simulink model "sim_4_newnew"  (R2015b)
settings: Solver=ode45  StartTime=0  StopTime=700  FixedStep=1e-3  RelTol=1e-4
undefined symbols (not defined in the file or in its folder): A, alpha_nc, alpha_nw, B, currentCoeffMatrix, D, E, f, H, h, K2, K3, K4, Kd_surge, Kd_sway, Kd_yaw, Ki_surge, Ki_sway, Ki_yaw, Kp_surge, Kp_sway, Kp_yaw, M_inverse, mu, N_freq, P0, Par, phi, Q, R, S, Sim, T, T_pinv, TA_sampling_time, thrusterPositionX, thrusterPositionY, thrusters, thrustersInitialAlpha, U_mean_c, U_mean_w, windCoeffMatrix, x0
libraries: simulink_extras x15, simulink x10, marine_gnc x5
(part 1 of 2)
settings Model: Creator=torstebo  LastModifiedBy=ShivJeet
settings SolverCC: MaxConsecutiveMinStep=3  SolverJacobianMethodControl=FullPerturbation  ZeroCrossControl=DisableAll  ZeroCrossAlgorithm=Adaptive
settings DataIOCC: Decimation=10  InitialState=xFinal  LimitDataPoints=off  SaveFormat=StructureWithTime  SaveOutput=off  InspectSignalLogs=on  VisualizeSimOutput=off  SaveTime=off
settings OptimizationCC: AccelVerboseBuild=on
settings DebuggingCC: AlgebraicLoopMsg=error  UnderspecifiedInitializationDetection=Classic  MergeDetectMultiDrivingBlocksExec=none  SolverPrmCheckMsg=warning  StateNameClashWarn=warning
settings HardwareCC: ProdBitPerPointer=32  ProdLargestAtomicFloat=None  ProdIntDivRoundTo=Undefined  ProdEndianess=Unspecified  ProdWordSize=32  ProdHWDeviceType=32-bit Generic
settings GRTTargetCC: GeneratePreprocessorConditionals=Disable all
settings ConfigComp: CovModelRefEnable=Off  CovSFcnEnable=off

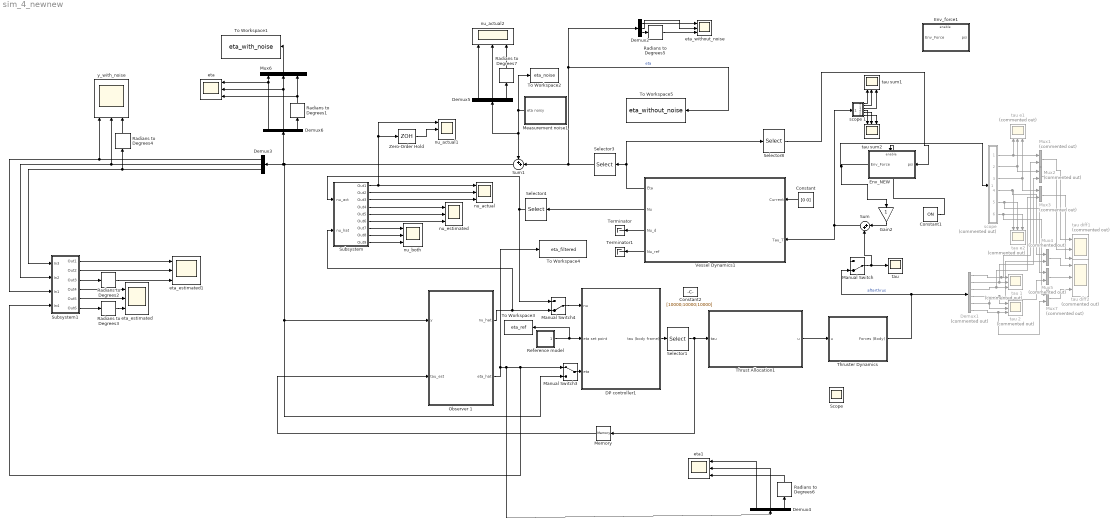
== system sim_4_newnew ==
  Constant : Constant  Value=[0 0]
  Constant1 : Constant  Value=ON
  Constant2 : Constant  Value=[10000;10000;10000]
  DP controller1 : Subsystem
  Demux1 : Demux  Commented=on  Outputs=6
  Demux{2..6} (5 alike) : Demux  Outputs=3
  Env_NEW : Subsystem
  Env_force1 : Subsystem
  Gain2 : Gain
  Manual Switch : ManualSwitch  CurrentSetting=0
  Manual Switch3 : ManualSwitch
  Manual Switch4 : ManualSwitch  CurrentSetting=0
  Measurement noise1 : Subsystem  mask{noise=on}
      mask prompts: noise "Use measurement noise"
  Memory : Memory  InheritSampleTime=on
  Mux{1..5,7} (6 alike) : Mux  Commented=on  Inputs=2
  Mux6 : Mux  Inputs=3
  Observer 1 : Subsystem
  Radians to Degrees{1..7} (7 alike) : simulink_extras/Transformations/Radians to Degrees
  Reference model : Subsystem
  Scope : Scope
  Selector1 : Selector  InputPortWidth=6  IndexOptions=Index vector (dialog)  Indices=[1 2 6]  OutputSizes=1
  Selector3 : Selector  InputPortWidth=6  IndexOptions=Index vector (dialog)  Indices=[1 2 6]  OutputSizes=1
  Selector4 : Selector  InputPortWidth=6  IndexOptions=Index vector (dialog)  Indices=[1 2 6]  OutputSizes=1
  Selector8 : Selector  InputPortWidth=6  IndexOptions=Index vector (dialog)  Indices=[6]  OutputSizes=1
  Subsystem : Subsystem
  Subsystem1 : Subsystem
  Sum : Sum  Inputs=|++
  Sum1 : Sum  Inputs=++|
  Terminator : Terminator
  Terminator1 : Terminator
  Thrust Allocation1 : Subsystem
  Thruster Dynamics : Subsystem  SystemSampleTime=TA_sampling_time  mask{wt=2, thrusterfault=off}
      mask prompts: wt "Thrusters Time constant"; thrusterfault "Thruster #3 fault?"
  To Workspace1 : ToWorkspace  VariableName=eta_with_noise  SaveFormat=Timeseries  SampleTime=-1
  To Workspace2 : ToWorkspace  VariableName=eta_noise  SaveFormat=Timeseries  SampleTime=-1
  To Workspace3 : ToWorkspace  VariableName=eta_ref  SaveFormat=Timeseries  SampleTime=-1
  To Workspace4 : ToWorkspace  VariableName=eta_filtered  SaveFormat=Timeseries  SampleTime=-1
  To Workspace5 : ToWorkspace  VariableName=eta_without_noise  SaveFormat=Timeseries  SampleTime=-1
  Vessel Dynamics1 : Subsystem
      mask Display:
      | image(imread('Files/supply.jpg'))
      | color('black'); port_label('output', 1, 'eta')
      | color('black'); port_label('output', 2, 'nu')
      | color('black'); port_label('output', 3, 'nu_d')
      | color('black'); port_label('output', 4, 'nu_ref')
      | color('black'); port_label('input', 1, 'nu_c')
      | color('black'); port_label('input', 2, 'tau')
  Zero-Order Hold : ZeroOrderHold  SampleTime=0.1
  eta : Scope  NumInputPorts=3
  eta1 : Scope  NumInputPorts=3
  eta_estimated : Scope  NumInputPorts=3
  eta_estimated1 : Scope  NumInputPorts=3
  eta_without_noise : Scope  NumInputPorts=3
  nu_actual : Scope  NumInputPorts=3
  nu_actual1 : Scope  NumInputPorts=3
  nu_actual2 : Scope  NumInputPorts=3
  "nu_both " : Scope  NumInputPorts=3
  nu_estimated : Scope  NumInputPorts=3
  "scope " : Subsystem  Commented=on
  scope 1 : Subsystem
  "tau " : Scope
  tau 1 : Scope  Commented=on  NumInputPorts=3
  tau 2 : Scope  Commented=on  NumInputPorts=3
  tau diff1 : Scope  Commented=on  NumInputPorts=3
  tau diff2 : Scope  Commented=on  NumInputPorts=3
  tau e1 : Scope  Commented=on  NumInputPorts=3
  tau e2 : Scope  Commented=on  NumInputPorts=3
  tau sum1 : Scope  NumInputPorts=3
  tau sum2 : Scope  NumInputPorts=3
  y_with_noise : Scope  NumInputPorts=3
  wires:
  Vessel Dynamics1/2(Nu) -> Selector4/1
  Constant/1 -> Vessel Dynamics1/1(Current)
  Reference model/1(Set-point) -> DP controller1/2(eta set point), To Workspace3/1
  Vessel Dynamics1/3(Nu_d) -> Terminator/1
  Thrust Allocation1/1(u) -> Thruster Dynamics/1(u)
  Vessel Dynamics1/4(Nu_ref) -> Terminator1/1
  Thruster Dynamics/1(Forces (Body)) -> Manual Switch/2, Demux1/1  "afterthrus"
  Demux6/3 -> Radians to Degrees1/1
  Radians to Degrees1/1 -> eta/3, Mux6/3
  Demux6/2 -> eta/2, Mux6/2
  Demux6/1 -> eta/1, Mux6/1
  Mux6/1 -> To Workspace1/1
  Vessel Dynamics1/1(Eta) -> Selector3/1, Selector8/1
  Selector8/1 -> Env_NEW/1(psi)
  Sum/1 -> scope 1/1(In1), Vessel Dynamics1/2(Tau_T)
  Manual Switch/1 -> "tau "/1, Sum/2
  Demux1/1 -> Mux1/2, tau 1/1
  Demux1/2 -> Mux2/2, tau 1/2
  Demux1/3 -> Mux3/2, tau 1/3
  Demux1/4 -> Mux4/2, tau 2/1
  Demux1/5 -> tau 2/2, Mux5/2
  Demux1/6 -> Mux7/2, tau 2/3
  Env_NEW/1(Env_Force) -> Gain2/1, "scope "/1(In1)
  "scope "/1(Out1) -> Mux1/1, tau e1/1
  "scope "/3(Out3) -> Mux3/1, tau e1/3
  "scope "/4(Out4) -> Mux4/1, tau e2/1
  "scope "/5(Out5) -> Mux5/1, tau e2/2
  "scope "/6(Out6) -> Mux7/1, tau e2/3
  scope 1/1(Out1) -> tau sum1/1
  scope 1/2(Out2) -> tau sum1/2
  scope 1/3(Out3) -> tau sum1/3
  scope 1/4(Out4) -> tau sum2/1
  scope 1/5(Out5) -> tau sum2/2
  scope 1/6(Out6) -> tau sum2/3
  Mux1/1 -> tau diff1/1
  "scope "/2(Out2) -> tau e1/2, Mux2/1
  Mux2/1 -> tau diff1/2
  Mux3/1 -> tau diff1/3
  Mux4/1 -> tau diff2/1
  Mux5/1 -> tau diff2/2
  Mux7/1 -> tau diff2/3
  Demux2/1 -> eta_without_noise/1
  Demux2/2 -> eta_without_noise/2
  Demux3/1 -> Subsystem1/3(In1), y_with_noise/1
  Demux3/2 -> Subsystem1/2(In2), y_with_noise/2
  Demux3/3 -> Subsystem1/1(In3), Radians to Degrees4/1
  Manual Switch4/1 -> DP controller1/1(nu)
  Observer 1/2(eta_hat) -> To Workspace4/1, Demux4/1, Subsystem1/4(In4), Manual Switch3/1
  Manual Switch3/1 -> DP controller1/3(eta)
  Selector4/1 -> Manual Switch4/1, Subsystem/1(nu_act)
  Sum1/1 -> Demux6/1, Demux3/1, Manual Switch3/2, Observer 1/1(y)
  Selector3/1 -> Demux2/1, To Workspace5/1, Sum1/2  "eta"
  Memory/1 -> Observer 1/2(tau_est)
  Subsystem/1(Out1) -> Zero-Order Hold/1, nu_actual1/1, nu_actual/1
  Subsystem/2(Out2) -> nu_actual/2
  Subsystem/3(Out3) -> nu_actual/3
  Subsystem/4(Out4) -> nu_estimated/1
  Subsystem/5(Out5) -> nu_estimated/2
  Subsystem/6(Out6) -> nu_estimated/3
  Subsystem/7(Out7) -> "nu_both "/1
  Subsystem/8(Out8) -> "nu_both "/2
  Subsystem/9(Out9) -> "nu_both "/3
  Subsystem1/1(Out1) -> eta_estimated1/1
  Subsystem1/2(Out2) -> eta_estimated1/2
  Subsystem1/3(Out3) -> Radians to Degrees2/1
  Subsystem1/4(Out4) -> eta_estimated/1
  Subsystem1/5(Out5) -> eta_estimated/2
  Subsystem1/6(Out6) -> Radians to Degrees3/1
  Radians to Degrees2/1 -> eta_estimated1/3
  Radians to Degrees3/1 -> eta_estimated/3
  Radians to Degrees4/1 -> y_with_noise/3
  Gain2/1 -> Sum/1
  Demux2/3 -> Radians to Degrees5/1
  Radians to Degrees5/1 -> eta_without_noise/3
  Demux4/3 -> Radians to Degrees6/1
  Radians to Degrees6/1 -> eta1/3
  Demux4/2 -> eta1/2
  Demux4/1 -> eta1/1
  Constant1/1 -> Env_NEW/Enable
  Observer 1/1(nu_hat) -> Subsystem/2(nu_hat), Manual Switch4/2
  Zero-Order Hold/1 -> nu_actual1/2
  Demux5/3 -> Radians to Degrees7/1
  Demux5/1 -> nu_actual2/1
  Measurement noise1/1(eta noisy) -> Demux5/1, Sum1/1, To Workspace2/1
  Demux5/2 -> nu_actual2/2
  Radians to Degrees7/1 -> nu_actual2/3
  DP controller1/1(tau (body frame)) -> Selector1/1
  Selector1/1 -> Thrust Allocation1/1(tau), Memory/1

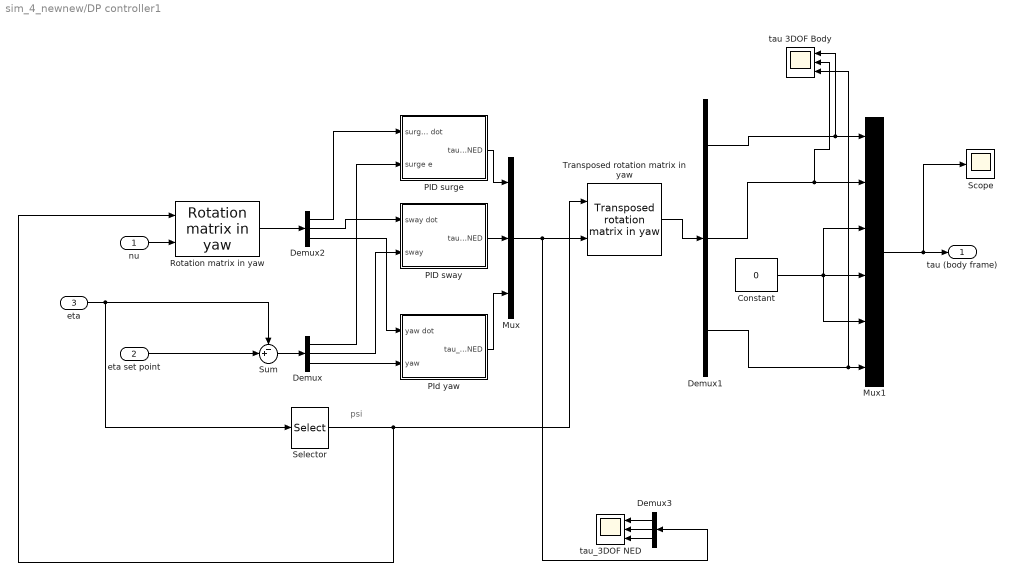
== system sim_4_newnew/DP controller1 ==
  note: psi
  nu : Inport
  eta set point : Inport  Port=2
  eta : Inport  Port=3
  Constant : Constant  Value=0
  Demux{,1..3} (4 alike) : Demux  Outputs=3
  Mux : Mux  Inputs=3
  Mux1 : Mux  Inputs=6
  PID surge : Subsystem
  PID sway : Subsystem
  "PId yaw " : Subsystem
  "Rotation matrix in yaw " : marine_gnc/Models/ Kinematics/Rotation matrix in yaw 
  Scope : Scope
  Selector : Selector  InputPortWidth=3  IndexOptions=Index vector (dialog)  Indices=3  OutputSizes=1
  Sum : Sum  Inputs=-+|
  Transposed rotation matrix in yaw : marine_gnc/Models/ Kinematics/Transposed rotation  matrix in yaw
  tau 3DOF Body : Scope  NumInputPorts=3
  tau_3DOF NED : Scope  NumInputPorts=3
  tau (body frame) : Outport
  wires:
  Sum/1 -> Demux/1
  eta/1 -> Sum/1, Selector/1
  eta set point/1 -> Sum/2
  Demux2/1 -> PID surge/1(surge dot)
  Demux/1 -> PID surge/2(surge e)
  Demux2/2 -> PID sway/1(sway dot)
  Demux2/3 -> "PId yaw "/1(yaw dot)
  Demux/2 -> PID sway/2(sway)
  Demux/3 -> "PId yaw "/2(yaw)
  "PId yaw "/1(tau_yaw_NED) -> Mux/3
  PID surge/1(tau_surge_NED) -> Mux/1
  PID sway/1(tau_sway_NED) -> Mux/2
  nu/1 -> "Rotation matrix in yaw "/2
  Selector/1 -> Transposed rotation matrix in yaw/1, "Rotation matrix in yaw "/1
  "Rotation matrix in yaw "/1 -> Demux2/1
  Constant/1 -> Mux1/3, Mux1/4, Mux1/5
  Transposed rotation matrix in yaw/1 -> Demux1/1
  Demux1/1 -> tau 3DOF Body/1, Mux1/1
  Demux1/2 -> tau 3DOF Body/2, Mux1/2
  Demux1/3 -> tau 3DOF Body/3, Mux1/6
  Mux1/1 -> Scope/1, tau (body frame)/1
  Demux3/1 -> tau_3DOF NED/1
  Demux3/2 -> tau_3DOF NED/2
  Demux3/3 -> tau_3DOF NED/3
  Mux/1 -> Transposed rotation matrix in yaw/2, Demux3/1

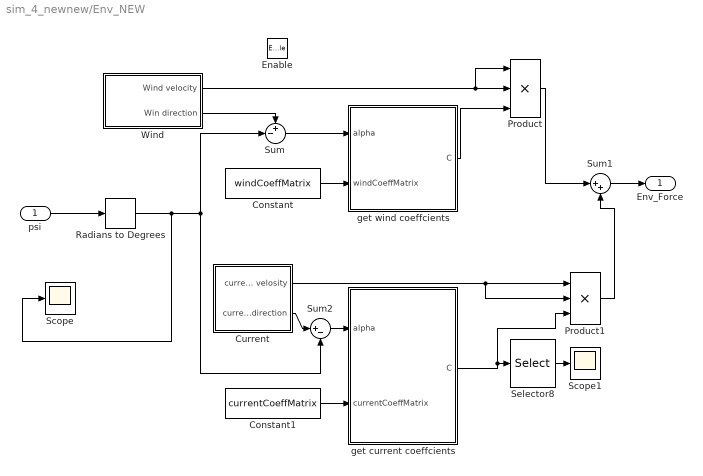
== system sim_4_newnew/Env_NEW ==
  psi : Inport
  Enable : EnablePort
  Constant : Constant  Value=windCoeffMatrix
  Constant1 : Constant  Value=currentCoeffMatrix
  Current : Subsystem
  Product : Product  Inputs=3  RndMeth=Zero
  Product1 : Product  Inputs=3  RndMeth=Zero
  Radians to Degrees : simulink_extras/Transformations/Radians to Degrees
  Scope : Scope
  Scope1 : Scope
  Selector8 : Selector  InputPortWidth=6  IndexOptions=Index vector (dialog)  Indices=[2]  OutputSizes=1
  Sum : Sum  Inputs=+-|
  Sum1 : Sum  Inputs=|++
  Sum2 : Sum  Inputs=|+-
  Wind : Subsystem
  get current coeffcients : MATLAB Function  TreatAsAtomicUnit=on
  get wind coeffcients : MATLAB Function  TreatAsAtomicUnit=on
  Env_Force : Outport
  wires:
  Wind/1(Wind velocity) -> Product/1, Product/2
  Wind/2(Win direction) -> Sum/1
  psi/1 -> Radians to Degrees/1
  Sum1/1 -> Env_Force/1
  Current/1(current velosity) -> Product1/2, Product1/1
  Radians to Degrees/1 -> Scope/1, Sum/2, Sum2/2
  Current/2(current direction) -> Sum2/1
  Sum2/1 -> get current coeffcients/1(alpha)
  get current coeffcients/1(C) -> Product1/3, Selector8/1
  Sum/1 -> get wind coeffcients/1(alpha)
  get wind coeffcients/1(C) -> Product/3
  Product1/1 -> Sum1/2
  Product/1 -> Sum1/1
  Selector8/1 -> Scope1/1
  Constant/1 -> get wind coeffcients/2(windCoeffMatrix)
  Constant1/1 -> get current coeffcients/2(currentCoeffMatrix)

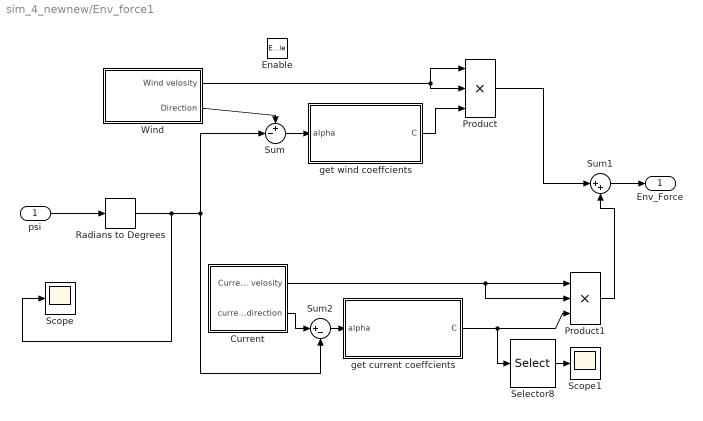
== system sim_4_newnew/Env_force1 ==
  psi : Inport
  Enable : EnablePort
  Current : Subsystem
  Product : Product  Inputs=3  RndMeth=Zero
  Product1 : Product  Inputs=3  RndMeth=Zero
  Radians to Degrees : simulink_extras/Transformations/Radians to Degrees
  Scope : Scope
  Scope1 : Scope
  Selector8 : Selector  InputPortWidth=6  IndexOptions=Index vector (dialog)  Indices=[2]  OutputSizes=1
  Sum : Sum  Inputs=+-|
  Sum1 : Sum  Inputs=|++
  Sum2 : Sum  Inputs=|+-
  Wind : Subsystem
  get current coeffcients : MATLAB Function  TreatAsAtomicUnit=on
  get wind coeffcients : MATLAB Function  TreatAsAtomicUnit=on
  Env_Force : Outport
  wires:
  Wind/1(Wind velosity) -> Product/1, Product/2
  Wind/2(Direction) -> Sum/1
  psi/1 -> Radians to Degrees/1
  Sum1/1 -> Env_Force/1
  Current/1(Current velosity) -> Product1/2, Product1/1
  Radians to Degrees/1 -> Scope/1, Sum/2, Sum2/2
  Current/2(current direction) -> Sum2/1
  Sum2/1 -> get current coeffcients/1(alpha)
  get current coeffcients/1(C) -> Selector8/1, Product1/3
  Sum/1 -> get wind coeffcients/1(alpha)
  get wind coeffcients/1(C) -> Product/3
  Product1/1 -> Sum1/2
  Product/1 -> Sum1/1
  Selector8/1 -> Scope1/1

== system sim_4_newnew/Measurement noise1 ==
  Band-Limited White Noise : simulink/Sources/Band-Limited White Noise  Cov="[0.003  0.003  0.0001]"  Ts=1/10  seed=[23341 10000 89564]
  Demux : Demux  Outputs=3
  Gain : Gain  Gain=noise
  Mux : Mux  Inputs=3
  Transfer Fcn : TransferFcn  Numerator=[10]  Denominator=[1 10]
  Transfer Fcn1 : TransferFcn  Numerator=[10]  Denominator=[1 10]
  Transfer Fcn2 : TransferFcn  Numerator=[10]  Denominator=[1 10]
  eta noisy : Outport
  wires:
  Gain/1 -> Demux/1
  Demux/3 -> Transfer Fcn2/1
  Demux/2 -> Transfer Fcn/1
  Demux/1 -> Transfer Fcn1/1
  Band-Limited White Noise/1 -> Gain/1
  Transfer Fcn2/1 -> Mux/3
  Transfer Fcn/1 -> Mux/2
  Transfer Fcn1/1 -> Mux/1
  Mux/1 -> eta noisy/1

== system sim_4_newnew/Observer 1 ==
  note: Fossen p.296
  note: Fossen p.312
  y : Inport
  tau_est : Inport  Port=2  PortDimensions=[3 1]
  Constant : Constant  Value=OFF
  Constant1 : Constant  Value=ON
  Demux : Demux  Outputs=6
  Extended Kalman Filter : Subsystem
  Manual Switch : ManualSwitch  CurrentSetting=0
  Mux : Mux  Inputs=2
  Mux2 : Mux  Inputs=3
  Mux3 : Mux  Inputs=3
  Nonlinear DP observer  using Compass and GNSS : Subsystem
  nu_hat : Outport
  eta_hat : Outport  Port=2
  wires:
  tau_est/1 -> Extended Kalman Filter/2(tau_est), Nonlinear DP observer  using Compass and GNSS/2("tau_est ")
  Nonlinear DP observer  using Compass and GNSS/1(eta_hat) -> Mux/1
  Nonlinear DP observer  using Compass and GNSS/2(nu_hat) -> Mux/2
  Demux/6 -> Mux2/3
  Demux/5 -> Mux2/2
  Demux/4 -> Mux2/1
  Demux/1 -> Mux3/1
  Demux/2 -> Mux3/2
  Demux/3 -> Mux3/3
  Mux3/1 -> eta_hat/1
  Mux2/1 -> nu_hat/1
  y/1 -> Extended Kalman Filter/1(y), Nonlinear DP observer  using Compass and GNSS/1(y)
  Constant/1 -> Nonlinear DP observer  using Compass and GNSS/Enable
  Manual Switch/1 -> Demux/1
  Mux/1 -> Manual Switch/1
  Extended Kalman Filter/1(eta_hat and nu_hat) -> Manual Switch/2
  Constant1/1 -> Extended Kalman Filter/Enable

== system sim_4_newnew/Reference model ==
  Mux : Mux  Inputs=3
  Sp_surge : Constant  Value=10*1  VectorParams1D=off
  Sp_sway : Constant  Value=2*1
  Sp_yaw : Constant  Value=pi/2
  Transfer Fcn1 : TransferFcn  Numerator=[0.05]  Denominator=[1 0.05]
  Transfer Fcn2 : TransferFcn  Numerator=[0.01]  Denominator=[1 0.01]
  Transfer Fcn3 : TransferFcn  Numerator=[0.05]  Denominator=[1 0.05]
  Set-point : Outport
  wires:
  Mux/1 -> Set-point/1
  Transfer Fcn1/1 -> Mux/1
  Transfer Fcn2/1 -> Mux/2
  Transfer Fcn3/1 -> Mux/3
  Sp_surge/1 -> Transfer Fcn1/1
  Sp_sway/1 -> Transfer Fcn2/1
  Sp_yaw/1 -> Transfer Fcn3/1

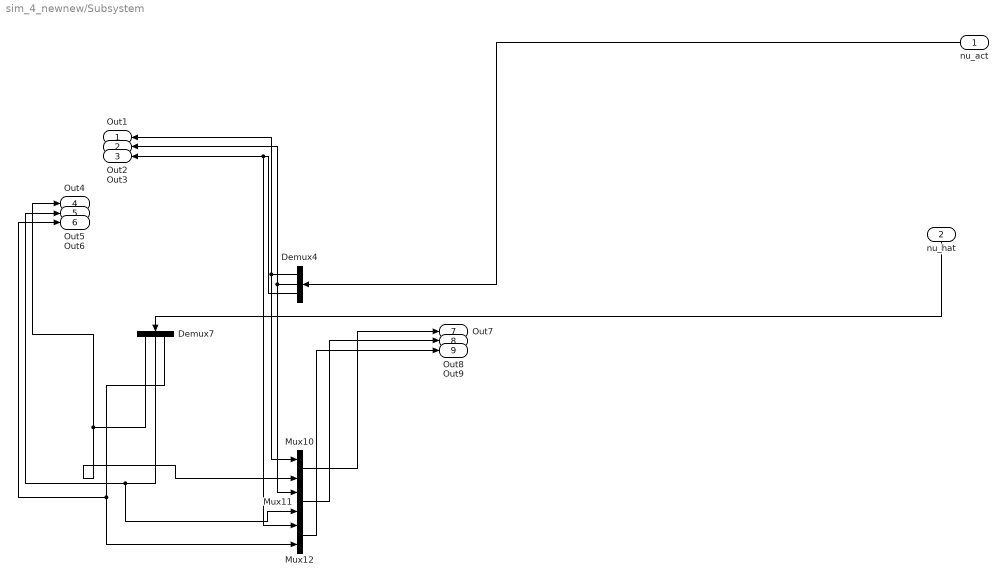
== system sim_4_newnew/Subsystem ==
  nu_act : Inport
  nu_hat : Inport  Port=2
  Demux4 : Demux  Outputs=3
  Demux7 : Demux  Outputs=3
  Mux10 : Mux  Inputs=2
  Mux11 : Mux  Inputs=2
  Mux12 : Mux  Inputs=2
  Out1 : Outport
  Out2 : Outport  Port=2
  Out3 : Outport  Port=3
  Out4 : Outport  Port=4
  Out5 : Outport  Port=5
  Out6 : Outport  Port=6
  Out7 : Outport  Port=7
  Out8 : Outport  Port=8
  Out9 : Outport  Port=9
  wires:
  nu_act/1 -> Demux4/1
  nu_hat/1 -> Demux7/1
  Demux4/1 -> Out1/1, Mux10/1
  Demux4/3 -> Out3/1, Mux12/1
  Mux10/1 -> Out7/1
  Demux4/2 -> Out2/1, Mux11/1
  Mux11/1 -> Out8/1
  Mux12/1 -> Out9/1
  Demux7/1 -> Mux10/2, Out4/1
  Demux7/2 -> Out5/1, Mux11/2
  Demux7/3 -> Out6/1, Mux12/2

== system sim_4_newnew/Subsystem1 ==
  In3 : Inport
  In2 : Inport  Port=2
  In1 : Inport  Port=3
  In4 : Inport  Port=4
  Demux5 : Demux  Outputs=3
  Mux : Mux  Inputs=2
  Mux8 : Mux  Inputs=2
  Mux9 : Mux  Inputs=2
  Out1 : Outport
  Out2 : Outport  Port=2
  Out3 : Outport  Port=3
  Out4 : Outport  Port=4
  Out5 : Outport  Port=5
  Out6 : Outport  Port=6
  wires:
  In2/1 -> Mux8/1
  In4/1 -> Demux5/1
  In3/1 -> Mux9/1
  In1/1 -> Mux/1
  Demux5/1 -> Out4/1, Mux/2
  Demux5/2 -> Out5/1, Mux8/2
  Demux5/3 -> Out6/1, Mux9/2
  Mux9/1 -> Out3/1
  Mux/1 -> Out1/1
  Mux8/1 -> Out2/1

== system sim_4_newnew/Thrust Allocation1 ==
  tau : Inport
  Gain : Gain  Gain=T_pinv  Multiplication=Matrix(K*u) (u vector)
  u : Outport
  wires:
  tau/1 -> Gain/1
  Gain/1 -> u/1

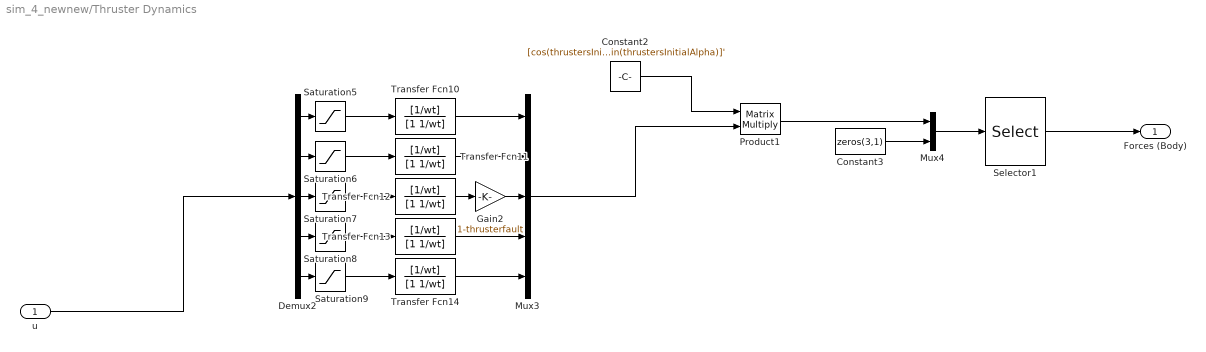
== system sim_4_newnew/Thruster Dynamics ==
  u : Inport  PortDimensions=[5 1]
  Constant2 : Constant  Value=[cos(thrustersInitialAlpha) sin(thrustersInitialAlpha) -thrusterPositionY.*cos(thrustersInitialAlpha)+thrusterPositionX.*sin(thrustersInitialAlpha)]'
  Constant3 : Constant  Value=zeros(3,1)
  Demux2 : Demux  Outputs=5
  Gain2 : Gain  Gain=1-thrusterfault
  Mux3 : Mux  Inputs=5
  Mux4 : Mux  Inputs=2
  Product1 : Product  Multiplication=Matrix(*)
  Saturation5 : Saturate  UpperLimit=thrusters(1).rated_thrust  LowerLimit=-thrusters(1).rated_thrust
  Saturation6 : Saturate  UpperLimit=thrusters(2).rated_thrust  LowerLimit=-thrusters(2).rated_thrust
  Saturation7 : Saturate  UpperLimit=thrusters(3).rated_thrust  LowerLimit=-thrusters(3).rated_thrust
  Saturation8 : Saturate  UpperLimit=thrusters(4).rated_thrust  LowerLimit=-thrusters(4).rated_thrust
  Saturation9 : Saturate  UpperLimit=thrusters(5).rated_thrust  LowerLimit=-thrusters(5).rated_thrust
  Selector1 : Selector  InputPortWidth=6  IndexOptions=Index vector (dialog)  Indices=[1 2 4 5 6 3]  OutputSizes=1
  Transfer Fcn{10..14} (5 alike) : TransferFcn  Numerator=[1/wt]  Denominator=[1 1/wt]
  Forces (Body) : Outport
  wires:
  Selector1/1 -> Forces (Body)/1
  Constant2/1 -> Product1/1
  Product1/1 -> Mux4/1
  Saturation5/1 -> Transfer Fcn10/1
  Demux2/1 -> Saturation5/1
  Demux2/2 -> Saturation6/1
  Saturation6/1 -> Transfer Fcn11/1
  Demux2/3 -> Saturation7/1
  Saturation7/1 -> Transfer Fcn12/1
  Demux2/4 -> Saturation8/1
  Saturation8/1 -> Transfer Fcn13/1
  Demux2/5 -> Saturation9/1
  Saturation9/1 -> Transfer Fcn14/1
  u/1 -> Demux2/1
  Transfer Fcn10/1 -> Mux3/1
  Transfer Fcn11/1 -> Mux3/2
  Transfer Fcn12/1 -> Gain2/1
  Transfer Fcn13/1 -> Mux3/4
  Transfer Fcn14/1 -> Mux3/5
  Mux4/1 -> Selector1/1
  Constant3/1 -> Mux4/2
  Gain2/1 -> Mux3/3
  Mux3/1 -> Product1/2

== system sim_4_newnew/Vessel Dynamics1 ==
  note: VESSEL MODULE
      | Consists of a WF and a LF module, which may be enabled or disabled in the Parameters file.
      | The LF and WFmotion components are written to the workspace for processing, and added for
      | use in the simulator.
  Current : Inport
  Tau_T : Inport  Port=2
  Vessel LF 6DOF : Subsystem
  Eta : Outport
  Nu : Outport  Port=2
  Nu_d : Outport  Port=3
  Nu_ref : Outport  Port=4
  wires:
  Current/1 -> Vessel LF 6DOF/2(Current_NED)
  Tau_T/1 -> Vessel LF 6DOF/1(External forces)  "Tau_T"
  Vessel LF 6DOF/1(Eta) -> Eta/1  "Eta_LF"
  Vessel LF 6DOF/2(Nu) -> Nu/1  "Nu_LF"
  Vessel LF 6DOF/3(Nu_d) -> Nu_d/1
  Vessel LF 6DOF/4(Nu_r) -> Nu_ref/1

== system sim_4_newnew/scope  ==
  In1 : Inport
  Demux2 : Demux  Outputs=6
  Out1 : Outport
  Out2 : Outport  Port=2
  Out3 : Outport  Port=3
  Out4 : Outport  Port=4
  Out5 : Outport  Port=5
  Out6 : Outport  Port=6
  wires:
  Demux2/2 -> Out2/1
  Demux2/1 -> Out1/1
  Demux2/5 -> Out5/1
  Demux2/4 -> Out4/1
  Demux2/6 -> Out6/1
  Demux2/3 -> Out3/1
  In1/1 -> Demux2/1

== system sim_4_newnew/scope 1 ==
  In1 : Inport
  Demux2 : Demux  Outputs=6
  Out1 : Outport
  Out2 : Outport  Port=2
  Out3 : Outport  Port=3
  Out4 : Outport  Port=4
  Out5 : Outport  Port=5
  Out6 : Outport  Port=6
  wires:
  Demux2/2 -> Out2/1
  Demux2/1 -> Out1/1
  Demux2/5 -> Out5/1
  Demux2/4 -> Out4/1
  Demux2/6 -> Out6/1
  Demux2/3 -> Out3/1
  In1/1 -> Demux2/1

== system sim_4_newnew/DP controller1/PID surge ==
  surge dot : Inport
  surge e : Inport  Port=2
  Gain2 : Gain  Gain=Ki_surge
  Integrator : Integrator
  KP : Gain  Gain=Kp_surge
  Kd : Gain  Gain=Kd_surge
  Sum : Sum  Inputs=|-++
  tau_surge_NED : Outport
  wires:
  surge dot/1 -> Kd/1
  surge e/1 -> KP/1, Integrator/1
  Integrator/1 -> Gain2/1
  Kd/1 -> Sum/1
  KP/1 -> Sum/2
  Gain2/1 -> Sum/3
  Sum/1 -> tau_surge_NED/1

== system sim_4_newnew/DP controller1/PID sway ==
  sway dot : Inport
  sway : Inport  Port=2
  Integrator : Integrator
  Kd : Gain  Gain=Kd_sway
  Ki : Gain  Gain=Ki_sway
  Kp : Gain  Gain=Kp_sway
  Sum : Sum  Inputs=|-++
  tau_sway_NED : Outport
  wires:
  sway dot/1 -> Kd/1
  sway/1 -> Kp/1, Integrator/1
  Integrator/1 -> Ki/1
  Kd/1 -> Sum/1
  Kp/1 -> Sum/2
  Ki/1 -> Sum/3
  Sum/1 -> tau_sway_NED/1

== system sim_4_newnew/DP controller1/PId yaw  ==
  yaw dot : Inport
  yaw : Inport  Port=2
  Gain : Gain  Gain=Kd_yaw
  Gain1 : Gain  Gain=Kp_yaw
  Gain2 : Gain  Gain=Ki_yaw
  Integrator : Integrator
  Sum : Sum  Inputs=|-++
  tau_yaw_NED : Outport
  wires:
  yaw dot/1 -> Gain/1
  yaw/1 -> Gain1/1, Integrator/1
  Integrator/1 -> Gain2/1
  Gain/1 -> Sum/1
  Gain1/1 -> Sum/2
  Gain2/1 -> Sum/3
  Sum/1 -> tau_yaw_NED/1

== system sim_4_newnew/Env_NEW/Current ==
  Divide : Product  Inputs=*/
  Fcn : Fcn  Expr=acos(u)
  MATLAB Function : MATLAB Function  TreatAsAtomicUnit=on
  Mux : Mux  Inputs=2
  Radians to Degrees : simulink_extras/Transformations/Radians to Degrees
  Scope{,1..2,4} (4 alike) : Scope  NumInputPorts=2
  Slowly-varying wind : Subsystem
  Sum : Sum  Inputs=++|
  Sum1 : Sum  Inputs=|++
  length : MATLAB Function  TreatAsAtomicUnit=on
  mean wind : Subsystem
  current velosity : Outport
  current direction : Outport  Port=2
  wires:
  Slowly-varying wind/1(SV_north) -> Scope2/1, Sum1/1
  mean wind/1(Mean_north) -> Sum1/2
  Slowly-varying wind/2(SV_east) -> Scope2/2, Scope1/1, Sum/1
  mean wind/2(Mean_east) -> Scope1/2, Sum/2
  Sum1/1 -> Divide/1, Mux/1
  Sum/1 -> Mux/2, Scope4/1, MATLAB Function/2(east)
  Mux/1 -> length/1(v)
  length/1(V) -> Divide/2, current velosity/1
  Divide/1 -> Fcn/1
  Fcn/1 -> Radians to Degrees/1
  MATLAB Function/1(alpha2) -> Scope/1, current direction/1
  Radians to Degrees/1 -> Scope/2, MATLAB Function/1(alpha1)

== system sim_4_newnew/Env_NEW/Wind ==
  note: |V|
  Divide : Product  Inputs=*/
  Fcn : Fcn  Expr=asin(u)
  Product : Product
  Product1 : Product
  Radians to Degrees : simulink_extras/Transformations/Radians to Degrees
  Scope : Scope
  Scope2 : Scope
  Slowly-varying wind + gust : Subsystem
  Sqrt : Sqrt  SaturateOnIntegerOverflow=on
  Sum : Sum  Inputs=++|
  Sum1 : Sum  Inputs=++|
  Sum2 : Sum  Inputs=+|+
  get the angle in the 1st and 2nd quadrant : MATLAB Function  TreatAsAtomicUnit=on
  mean wind : Subsystem
  Wind velocity : Outport
  Win direction : Outport  Port=2
  wires:
  Slowly-varying wind + gust/2(SV_east + gust) -> Sum/1
  mean wind/2(Mean_east) -> Sum/2
  Sum1/1 -> Product/1, Product/2, get the angle in the 1st and 2nd quadrant/2(north)  "U_north"
  Sum/1 -> Product1/2, Product1/1, Divide/1
  Sqrt/1 -> Divide/2, Wind velocity/1
  Radians to Degrees/1 -> Win direction/1, Scope/1
  get the angle in the 1st and 2nd quadrant/1(alpha2) -> Radians to Degrees/1
  Slowly-varying wind + gust/1(SV_north + gust) -> Sum1/2
  mean wind/1(Mean_north) -> Sum1/1
  Product/1 -> Sum2/1
  Product1/1 -> Sum2/2
  Sum2/1 -> Sqrt/1
  Divide/1 -> Fcn/1
  Fcn/1 -> Scope2/1, get the angle in the 1st and 2nd quadrant/1(alpha1)

== system sim_4_newnew/Env_force1/Current ==
  Divide : Product  Inputs=*/
  Fcn : Fcn  Expr=acos(u)
  MATLAB Function : MATLAB Function  TreatAsAtomicUnit=on
  Mux : Mux  Inputs=2
  Radians to Degrees : simulink_extras/Transformations/Radians to Degrees
  Scope{,1..2,4} (4 alike) : Scope  NumInputPorts=2
  Slowly-varying wind : Subsystem
  Sum : Sum  Inputs=++|
  Sum1 : Sum  Inputs=|++
  length : MATLAB Function  TreatAsAtomicUnit=on
  mean wind : Subsystem
  Current velosity : Outport
  current direction : Outport  Port=2
  wires:
  Slowly-varying wind/1(SV_north) -> Scope2/1, Sum1/1
  mean wind/1(Mean_north) -> Sum1/2
  Slowly-varying wind/2(SV_east) -> Scope2/2, Scope1/1, Sum/1
  mean wind/2(Mean_east) -> Scope1/2, Sum/2
  Sum1/1 -> Divide/1, Mux/1
  Sum/1 -> Mux/2, Scope4/1, MATLAB Function/2(east)
  Mux/1 -> length/1(v)
  length/1(V) -> Divide/2, Current velosity/1
  Divide/1 -> Fcn/1
  Fcn/1 -> Radians to Degrees/1
  MATLAB Function/1(alpha2) -> Scope/1, current direction/1
  Radians to Degrees/1 -> Scope/2, MATLAB Function/1(alpha1)

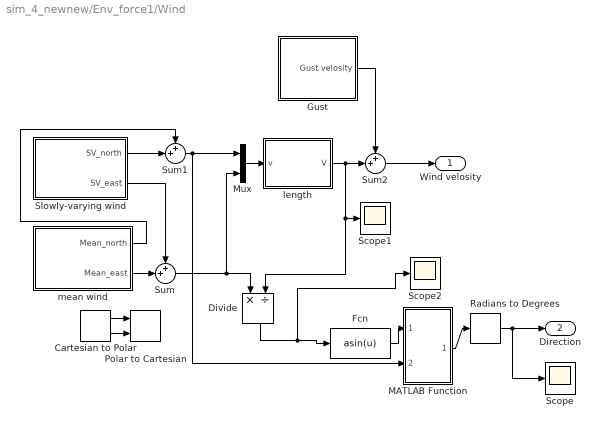
== system sim_4_newnew/Env_force1/Wind ==
  Cartesian to Polar : simulink_extras/Transformations/Cartesian to Polar
  Divide : Product  Inputs=*/
  Fcn : Fcn  Expr=asin(u)
  Gust : Subsystem
  MATLAB Function : MATLAB Function  TreatAsAtomicUnit=on
  Mux : Mux  Inputs=2
  Polar to Cartesian : simulink_extras/Transformations/Polar to Cartesian
  Radians to Degrees : simulink_extras/Transformations/Radians to Degrees
  Scope : Scope
  Scope1 : Scope
  Scope2 : Scope
  Slowly-varying wind : Subsystem
  Sum : Sum  Inputs=++|
  Sum1 : Sum  Inputs=++|
  Sum2 : Sum  Inputs=++|
  length : MATLAB Function  TreatAsAtomicUnit=on
  mean wind : Subsystem
  Wind velosity : Outport
  Direction : Outport  Port=2
  wires:
  Slowly-varying wind/2(SV_east) -> Sum/1
  mean wind/2(Mean_east) -> Sum/2
  Sum1/1 -> Mux/1, MATLAB Function/2(north)
  Sum/1 -> Mux/2, Divide/1
  Mux/1 -> length/1(v)
  length/1(V) -> Sum2/2, Scope1/1, Divide/2
  Divide/1 -> Fcn/1, Scope2/1
  Sum2/1 -> Wind velosity/1
  Radians to Degrees/1 -> Scope/1, Direction/1
  Gust/1(Gust velosity) -> Sum2/1
  Fcn/1 -> MATLAB Function/1(alpha1)
  MATLAB Function/1(alpha2) -> Radians to Degrees/1
  Slowly-varying wind/1(SV_north) -> Sum1/2
  mean wind/1(Mean_north) -> Sum1/1
  Cartesian to Polar/1 -> Polar to Cartesian/1
  Cartesian to Polar/2 -> Polar to Cartesian/2

== system sim_4_newnew/Observer 1/Extended Kalman Filter ==
  note: Used to update A
  y : Inport
  tau_est : Inport  Port=2
  Enable : EnablePort
  Constant : Constant  Value=h
  Constant1 : Constant  Value=M_inverse
  Constant2 : Constant  Value=Q
  Constant3 : Constant  Value=E
  Constant4 : Constant  Value=B
  Constant5 : Constant  Value=R
  Constant6 : Constant  Value=A
  Constant7 : Constant  Value=H
  Constant8 : Constant  Value=P0
  Constant9 : Constant  Value=x0
  Extended Kalman Filter : MATLAB Function  TreatAsAtomicUnit=on  SystemSampleTime=h
  eta_hat and nu_hat : Outport
  wires:
  y/1 -> Extended Kalman Filter/1(y)
  tau_est/1 -> Extended Kalman Filter/2(tau)
  Extended Kalman Filter/1(estimatedEtaAndNu) -> eta_hat and nu_hat/1
  Constant/1 -> Extended Kalman Filter/12(h)
  Constant1/1 -> Extended Kalman Filter/8(M_inverse)
  Constant2/1 -> Extended Kalman Filter/3(Q)
  Constant5/1 -> Extended Kalman Filter/4(R)
  Constant6/1 -> Extended Kalman Filter/7(A)
  Constant4/1 -> Extended Kalman Filter/9(B)
  Constant3/1 -> Extended Kalman Filter/10(E)
  Constant7/1 -> Extended Kalman Filter/11(H)
  Constant8/1 -> Extended Kalman Filter/6(P0)
  Constant9/1 -> Extended Kalman Filter/5(x0)

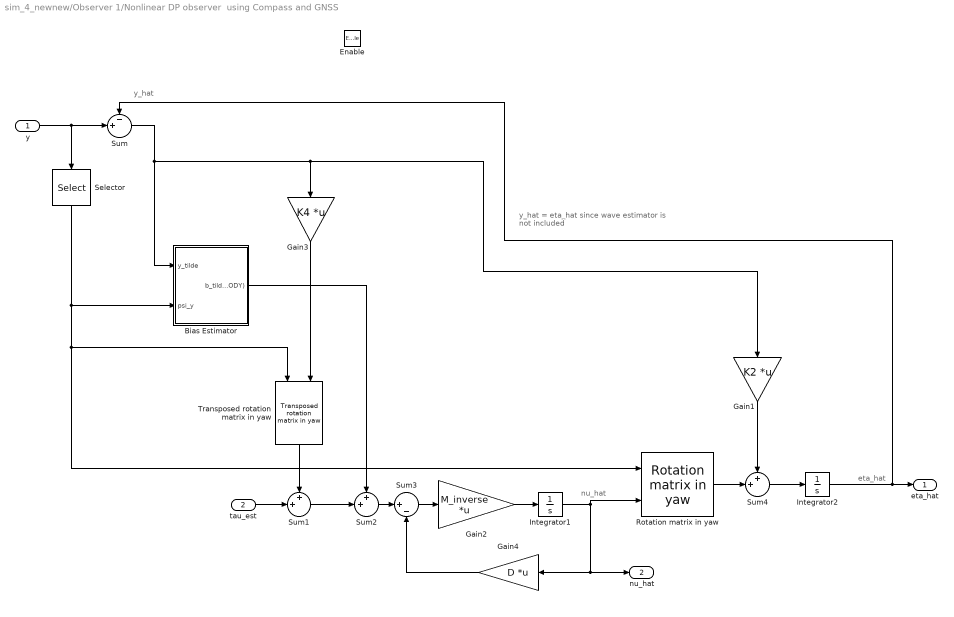
== system sim_4_newnew/Observer 1/Nonlinear DP observer  using Compass and GNSS ==
  note: y_hat
  note: y_hat = eta_hat
      | since wave estimator is not included
  note: eta_hat
  note: nu_hat
  y : Inport
  "tau_est " : Inport  Port=2
  Enable : EnablePort
  Bias Estimator : Subsystem
  Gain1 : Gain  Gain=K2  Multiplication=Matrix(K*u)
  Gain2 : Gain  Gain=M_inverse  Multiplication=Matrix(K*u)
  Gain3 : Gain  Gain=K4  Multiplication=Matrix(K*u)
  Gain4 : Gain  Gain=D  Multiplication=Matrix(K*u)
  Integrator1 : Integrator
  Integrator2 : Integrator
  "Rotation matrix in yaw " : marine_gnc/Models/ Kinematics/Rotation matrix in yaw 
  Selector : Selector  InputPortWidth=3  IndexOptions=Index vector (dialog)  Indices=[3]  OutputSizes=1
  Sum : Sum  Inputs=-+|
  Sum1 : Sum  Inputs=++|
  Sum2 : Sum  Inputs=++|
  Sum3 : Sum  Inputs=|+-
  Sum4 : Sum  Inputs=++|
  Transposed rotation matrix in yaw : marine_gnc/Models/ Kinematics/Transposed rotation  matrix in yaw
  eta_hat : Outport
  nu_hat : Outport  Port=2
  wires:
  y/1 -> Selector/1, Sum/2
  Sum/1 -> Gain1/1, Gain3/1, Bias Estimator/1(y_tilde)
  Selector/1 -> Transposed rotation matrix in yaw/1, "Rotation matrix in yaw "/1, Bias Estimator/2(psi_y)
  Gain3/1 -> Transposed rotation matrix in yaw/2
  Transposed rotation matrix in yaw/1 -> Sum1/1
  Bias Estimator/1(b_tilde (BODY)) -> Sum2/1
  Sum1/1 -> Sum2/2
  Sum2/1 -> Sum3/1
  Sum3/1 -> Gain2/1
  Gain2/1 -> Integrator1/1
  Gain4/1 -> Sum3/2
  Integrator1/1 -> nu_hat/1, Gain4/1, "Rotation matrix in yaw "/2
  Gain1/1 -> Sum4/1
  "Rotation matrix in yaw "/1 -> Sum4/2
  Sum4/1 -> Integrator2/1
  Integrator2/1 -> Sum/1, eta_hat/1
  "tau_est "/1 -> Sum1/2

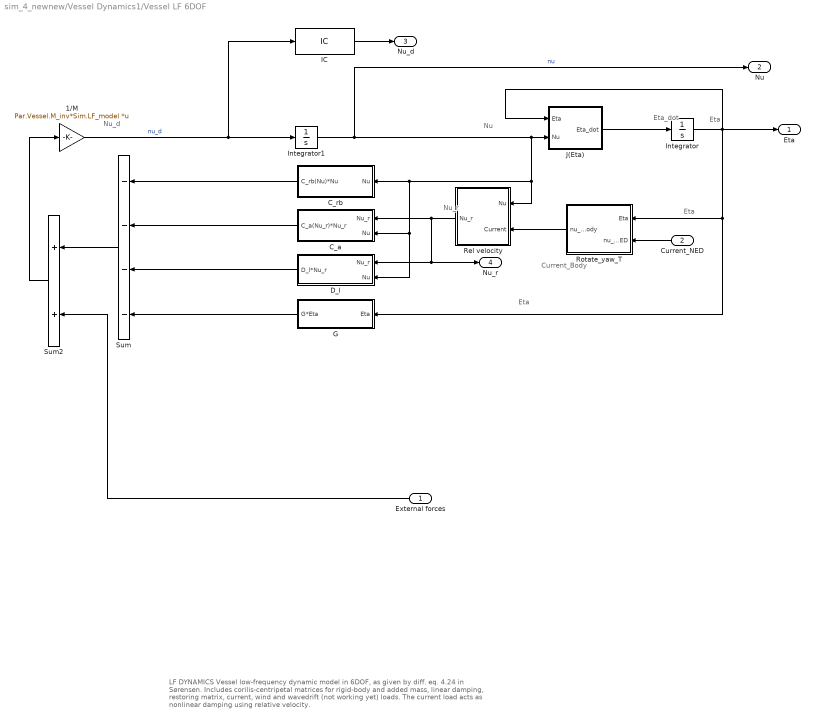
== system sim_4_newnew/Vessel Dynamics1/Vessel LF 6DOF ==
  note: Nu_d
  note: Nu
  note: Eta
  note: Current_Body
  note: Eta
  note: Nu_r
  note: Eta
  note: LF DYNAMICS
      | Vessel low-frequency dynamic model in 6DOF, as given by diff. eq. 4.24 in Sørensen.
      | Includes corilis-centripetal matrices for rigid-body and added mass, linear damping,
      | restoring matrix, current, wind and wavedrift (not working yet) loads. The current load
      | acts as nonlinear damping using relative velocity.
  note: Eta_dot
  External forces : Inport
  Current_NED : Inport  Port=2
  1/M : Gain  Gain=Par.Vessel.M_inv*Sim.LF_model  Multiplication=Matrix(K*u) (u vector)  SaturateOnIntegerOverflow=on  OutDataTypeStr=Inherit: Same as input  ParamDataTypeStr=Inherit: Same as input
  C_a : Subsystem
  C_rb : Subsystem
  D_l : Subsystem
      settings: MinAlgLoopOccurrences=on
  G : Subsystem
  IC : InitialCondition  Value=Sim.Nu_d_init
  Integrator : Integrator  InitialCondition=Sim.Eta_init
  Integrator1 : Integrator  InitialCondition=Sim.Nu_init
  J(Eta) : Subsystem
  Rel velocity : Subsystem
  Rotate_yaw_T : Subsystem
  Sum : Sum  Inputs=----  SaturateOnIntegerOverflow=on
  Sum2 : Sum  SaturateOnIntegerOverflow=on
  Eta : Outport
  Nu : Outport  Port=2
  Nu_d : Outport  Port=3
  Nu_r : Outport  Port=4
  wires:
  1/M/1 -> IC/1, Integrator1/1  "nu_d"
  J(Eta)/1(Eta_dot) -> Integrator/1
  Integrator/1 -> J(Eta)/1(Eta), Eta/1, Rotate_yaw_T/1(Eta), G/1(Eta)
  Integrator1/1 -> Nu/1, J(Eta)/2(Nu), Rel velocity/1(Nu), C_a/2(Nu), D_l/2(Nu), C_rb/1(Nu)  "nu"
  Current_NED/1 -> Rotate_yaw_T/2(nu_2D_NED)
  Rotate_yaw_T/1(nu_2D_body) -> Rel velocity/2(Current)
  Rel velocity/1(Nu_r) -> D_l/1(Nu_r), Nu_r/1, C_a/1(Nu_r)
  Sum/1 -> Sum2/1
  External forces/1 -> Sum2/2
  Sum2/1 -> 1/M/1
  C_rb/1(C_rb(Nu)*Nu) -> Sum/1
  C_a/1(C_a(Nu_r)*Nu_r) -> Sum/2
  D_l/1(D_l*Nu_r) -> Sum/3
  G/1(G*Eta) -> Sum/4
  IC/1 -> Nu_d/1

== system sim_4_newnew/Env_NEW/Current/Slowly-varying wind ==
  Band-Limited White Noise : simulink/Sources/Band-Limited White Noise  Cov=[0.00005]  Ts=20  seed=[23343]
  Band-Limited White Noise1 : simulink/Sources/Band-Limited White Noise  Cov=[0.00005]  Ts=20  seed=[23344]
  Constant : Constant  Value=mu
  Fcn : Fcn  Expr=sin(u)
  Fcn1 : Fcn  Expr=cos(u)
  Integrator : Integrator
  Product : Product  RndMeth=Zero
  Product1 : Product  RndMeth=Zero
  Product2 : Product  RndMeth=Zero
  Saturation : Saturate  UpperLimit=(5*pi)/180  LowerLimit=-(5*pi)/180
  Saturation1 : Saturate  UpperLimit=0.2  LowerLimit=-0.2
  Sum : Sum  Inputs=|+-
  Sum1 : Sum  Inputs=|++
  mean angel : Constant  Value=alpha_nc
  SV_north : Outport
  SV_east : Outport  Port=2
  wires:
  Band-Limited White Noise/1 -> Sum/1
  Sum/1 -> Integrator/1
  Integrator/1 -> Product/2, Saturation1/1
  Product/1 -> Sum/2
  Constant/1 -> Product/1
  Fcn/1 -> Product2/2
  Fcn1/1 -> Product1/2
  mean angel/1 -> Sum1/1
  Sum1/1 -> Fcn/1, Fcn1/1
  Saturation/1 -> Sum1/2
  Band-Limited White Noise1/1 -> Saturation/1
  Product1/1 -> SV_north/1
  Product2/1 -> SV_east/1
  Saturation1/1 -> Product1/1, Product2/1

== system sim_4_newnew/Env_NEW/Current/mean wind ==
  Constant : Constant  Value=U_mean_c
  Fcn : Fcn  Expr=sin(u)
  Fcn1 : Fcn  Expr=cos(u)
  Product1 : Product  RndMeth=Zero
  Product2 : Product  RndMeth=Zero
  meen wind : Constant  Value=alpha_nc
  Mean_north : Outport
  Mean_east : Outport  Port=2
  wires:
  Constant/1 -> Product1/1, Product2/1
  Fcn/1 -> Product2/2
  Fcn1/1 -> Product1/2
  Product1/1 -> Mean_north/1
  Product2/1 -> Mean_east/1
  meen wind/1 -> Fcn/1, Fcn1/1

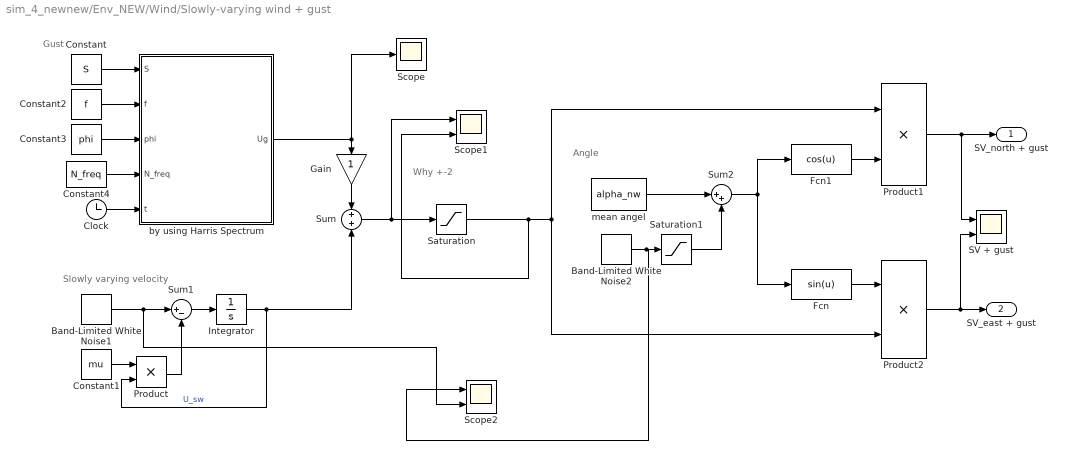
== system sim_4_newnew/Env_NEW/Wind/Slowly-varying wind + gust ==
  note: Gust
  note: Slowly varying velocity
  note: Angle
  note: Why +-2
  Band-Limited White Noise1 : simulink/Sources/Band-Limited White Noise  Cov=[0.005]  Ts=20  seed=[23341]
  Band-Limited White Noise2 : simulink/Sources/Band-Limited White Noise  Cov=[0.005]  Ts=20  seed=[23342]
  Clock : Clock
  Constant : Constant  Value=S
  Constant1 : Constant  Value=mu
  Constant2 : Constant  Value=f
  Constant3 : Constant  Value=phi
  Constant4 : Constant  Value=N_freq
  Fcn : Fcn  Expr=sin(u)
  Fcn1 : Fcn  Expr=cos(u)
  Gain : Gain
  Integrator : Integrator
  Product : Product  RndMeth=Zero
  Product1 : Product  RndMeth=Zero
  Product2 : Product  RndMeth=Zero
  SV + gust : Scope  NumInputPorts=2
  Saturation : Saturate  UpperLimit=2  LowerLimit=-2
  Saturation1 : Saturate  UpperLimit=(5*pi)/180  LowerLimit=-(5*pi)/180
  Scope : Scope
  Scope1 : Scope  NumInputPorts=2
  Scope2 : Scope  NumInputPorts=2
  Sum : Sum  Inputs=+|+
  Sum1 : Sum  Inputs=|+-
  Sum2 : Sum  Inputs=|++
  by using Harris Spectrum : MATLAB Function  TreatAsAtomicUnit=on  SystemSampleTime=1
  mean angel : Constant  Value=alpha_nw
  SV_north + gust : Outport
  SV_east + gust : Outport  Port=2
  wires:
  Fcn1/1 -> Product1/2
  Product1/1 -> SV + gust/1, SV_north + gust/1
  Product2/1 -> SV_east + gust/1, SV + gust/2
  Sum2/1 -> Fcn/1, Fcn1/1
  Integrator/1 -> Sum/2, Product/2  "U_sw"
  Saturation/1 -> Scope1/2, Product1/1, Product2/2
  Constant1/1 -> Product/1
  Sum1/1 -> Integrator/1
  Product/1 -> Sum1/2
  Band-Limited White Noise1/1 -> Scope2/2, Sum1/1
  mean angel/1 -> Sum2/1
  Saturation1/1 -> Sum2/2
  Band-Limited White Noise2/1 -> Scope2/1, Saturation1/1
  Fcn/1 -> Product2/1
  Constant/1 -> by using Harris Spectrum/1(S)
  Constant2/1 -> by using Harris Spectrum/2(f)
  Constant3/1 -> by using Harris Spectrum/3(phi)
  Constant4/1 -> by using Harris Spectrum/4(N_freq)
  by using Harris Spectrum/1(Ug) -> Gain/1, Scope/1
  Clock/1 -> by using Harris Spectrum/5(t)
  Sum/1 -> Scope1/1, Saturation/1
  Gain/1 -> Sum/1

== system sim_4_newnew/Env_NEW/Wind/mean wind ==
  Constant : Constant  Value=U_mean_w
  Fcn : Fcn  Expr=sin(u)
  Fcn1 : Fcn  Expr=cos(u)
  Product1 : Product  RndMeth=Zero
  Product2 : Product  RndMeth=Zero
  mean wind : Constant  Value=alpha_nw
  Mean_north : Outport
  Mean_east : Outport  Port=2
  wires:
  Constant/1 -> Product2/2, Product1/1
  Fcn1/1 -> Product1/2
  Product1/1 -> Mean_north/1
  mean wind/1 -> Fcn1/1, Fcn/1
  Fcn/1 -> Product2/1
  Product2/1 -> Mean_east/1

== system sim_4_newnew/Env_force1/Current/Slowly-varying wind ==
  Band-Limited White Noise : simulink/Sources/Band-Limited White Noise  Cov=[0.00005]  Ts=20  seed=[23341]
  Band-Limited White Noise1 : simulink/Sources/Band-Limited White Noise  Cov=[0.00005]  Ts=20  seed=[23341]
  Constant : Constant  Value=mu
  Fcn : Fcn  Expr=sin(u)
  Fcn1 : Fcn  Expr=cos(u)
  Integrator : Integrator
  Product : Product  RndMeth=Zero
  Product1 : Product  RndMeth=Zero
  Product2 : Product  RndMeth=Zero
  Saturation : Saturate  UpperLimit=(5*pi)/180  LowerLimit=-(5*pi)/180
  Sum : Sum  Inputs=|+-
  Sum1 : Sum  Inputs=|++
  mean angel : Constant  Value=alpha_nc
  SV_north : Outport
  SV_east : Outport  Port=2
  wires:
  Band-Limited White Noise/1 -> Sum/1
  Sum/1 -> Integrator/1
  Integrator/1 -> Product/2, Product1/1, Product2/1
  Product/1 -> Sum/2
  Constant/1 -> Product/1
  Fcn/1 -> Product2/2
  Fcn1/1 -> Product1/2
  mean angel/1 -> Sum1/1
  Sum1/1 -> Fcn/1, Fcn1/1
  Saturation/1 -> Sum1/2
  Band-Limited White Noise1/1 -> Saturation/1
  Product1/1 -> SV_north/1
  Product2/1 -> SV_east/1

== system sim_4_newnew/Env_force1/Current/mean wind ==
  Constant : Constant  Value=U_mean_c
  Fcn : Fcn  Expr=sin(u)
  Fcn1 : Fcn  Expr=cos(u)
  Product1 : Product  RndMeth=Zero
  Product2 : Product  RndMeth=Zero
  meen wind : Constant  Value=alpha_nc
  Mean_north : Outport
  Mean_east : Outport  Port=2
  wires:
  Constant/1 -> Product1/1, Product2/1
  Fcn/1 -> Product2/2
  Fcn1/1 -> Product1/2
  Product1/1 -> Mean_north/1
  Product2/1 -> Mean_east/1
  meen wind/1 -> Fcn/1, Fcn1/1

== system sim_4_newnew/Env_force1/Wind/Gust ==
  Band-Limited White Noise : simulink/Sources/Band-Limited White Noise  Cov=[0.1]  Ts=0.1  seed=[23341]
  Constant : Constant  Value=0
  Sine Wave Function : Sin  TimeSource=Use external signal  Frequency=100  SampleTime=0
  Terminator : Terminator
  Gust velosity : Outport
  wires:
  Band-Limited White Noise/1 -> Sine Wave Function/1
  Constant/1 -> Gust velosity/1
  Sine Wave Function/1 -> Terminator/1

== system sim_4_newnew/Env_force1/Wind/Slowly-varying wind ==
  Band-Limited White Noise : simulink/Sources/Band-Limited White Noise  Cov=[0.005]  Ts=20  seed=[23341]
  Band-Limited White Noise1 : simulink/Sources/Band-Limited White Noise  Cov=[0.005]  Ts=20  seed=[23341]
  Constant : Constant  Value=mu
  Fcn : Fcn  Expr=sin(u)
  Fcn1 : Fcn  Expr=cos(u)
  Integrator : Integrator
  Product : Product  RndMeth=Zero
  Product1 : Product  RndMeth=Zero
  Product2 : Product  RndMeth=Zero
  Saturation : Saturate  UpperLimit=(5*pi)/180  LowerLimit=-(5*pi)/180
  Scope : Scope  NumInputPorts=2
  Sum : Sum  Inputs=|+-
  Sum1 : Sum  Inputs=|++
  mean angel : Constant  Value=alpha_nw
  SV_north : Outport
  SV_east : Outport  Port=2
  wires:
  Band-Limited White Noise/1 -> Sum/1
  Sum/1 -> Integrator/1
  Integrator/1 -> Product/2, Product1/1, Product2/1
  Product/1 -> Sum/2
  Constant/1 -> Product/1
  Fcn/1 -> Product2/2
  Fcn1/1 -> Product1/2
  mean angel/1 -> Sum1/1
  Sum1/1 -> Fcn/1, Fcn1/1
  Saturation/1 -> Sum1/2
  Band-Limited White Noise1/1 -> Saturation/1
  Product1/1 -> Scope/1, SV_north/1
  Product2/1 -> Scope/2, SV_east/1

== system sim_4_newnew/Env_force1/Wind/mean wind ==
  Constant : Constant  Value=U_mean_w
  Fcn : Fcn  Expr=sin(u)
  Fcn1 : Fcn  Expr=cos(u)
  Product1 : Product  RndMeth=Zero
  Product2 : Product  RndMeth=Zero
  mean wind : Constant  Value=alpha_nw
  Mean_north : Outport
  Mean_east : Outport  Port=2
  wires:
  Constant/1 -> Product1/1, Product2/1
  Fcn/1 -> Product2/2
  Fcn1/1 -> Product1/2
  Product1/1 -> Mean_north/1
  Product2/1 -> Mean_east/1
  mean wind/1 -> Fcn/1, Fcn1/1

== system sim_4_newnew/Observer 1/Nonlinear DP observer  using Compass and GNSS/Bias Estimator ==
  y_tilde : Inport
  psi_y : Inport  Port=2
  Gain2 : Gain  Gain=K3  Multiplication=Matrix(K*u)
  Gain4 : Gain  Gain=inv(T)  Multiplication=Matrix(K*u)
  Integrator : Integrator
  Sum1 : Sum  Inputs=|+-
  Transposed rotation matrix in yaw : marine_gnc/Models/ Kinematics/Transposed rotation  matrix in yaw
  b_tilde (BODY) : Outport
  wires:
  Integrator/1 -> Gain4/1, Transposed rotation matrix in yaw/2
  Transposed rotation matrix in yaw/1 -> b_tilde (BODY)/1
  psi_y/1 -> Transposed rotation matrix in yaw/1
  y_tilde/1 -> Gain2/1
  Sum1/1 -> Integrator/1
  Gain4/1 -> Sum1/2
  Gain2/1 -> Sum1/1

== system sim_4_newnew/Vessel Dynamics1/Vessel LF 6DOF/C_a ==
  note: C_a
      | Coriolis-centripetal added mass force calculation using the S-function m2c_S.
      | This effect can be included/excluded from the Parameters file.
      | A choice of using absolute or relative vessel velocity is also given.
      | OS2002
  Nu_r : Inport
  Nu : Inport  Port=2
  C_a calculation : Subsystem  TreatAsAtomicUnit=on
  Enable Coriolis added mass force : Constant  Value=Sim.C_a
  Sim.Nu_r_C_a : Constant  Value=Sim.Nu_r_C_a
  Switch : Switch  Criteria=u2 > Threshold  SaturateOnIntegerOverflow=on
  C_a(Nu_r)*Nu_r : Outport
  wires:
  C_a calculation/1(F) -> C_a(Nu_r)*Nu_r/1
  Nu_r/1 -> Switch/1
  Nu/1 -> Switch/3
  Sim.Nu_r_C_a/1 -> Switch/2
  Switch/1 -> C_a calculation/1(Nu_r)
  Enable Coriolis added mass force/1 -> C_a calculation/Enable

== system sim_4_newnew/Vessel Dynamics1/Vessel LF 6DOF/C_rb ==
  note: C_rb
      | Coriolis-centripetal rigid-body force calculation using the S-function m2c_S.
      | This effect can be included/excluded from the Parameters file.
      | OS2002
  Nu : Inport
  C_rb Calculation : Subsystem  TreatAsAtomicUnit=on
  Enable Coriolis added mass force : Constant  Value=Sim.C_rb
  C_rb(Nu)*Nu : Outport
  wires:
  Nu/1 -> C_rb Calculation/1(Nu_r)
  Enable Coriolis added mass force/1 -> C_rb Calculation/Enable
  C_rb Calculation/1(F) -> C_rb(Nu)*Nu/1

== system sim_4_newnew/Vessel Dynamics1/Vessel LF 6DOF/D_l ==
  note: D_l
      | Linear damping, matrix formulation.
      | This effect can be included/excluded from the Parameters file.
      | A choice of using absolute or relative vessel velocity is also given.
      | OS2002
  Nu_r : Inport
  Nu : Inport  Port=2
  D_l : Gain  Gain=Par.Vessel.DL  Multiplication=Matrix(K*u)  SaturateOnIntegerOverflow=on  OutDataTypeStr=Inherit: Same as input  ParamDataTypeStr=Inherit: Same as input
  Include D_l : Gain  Gain=Sim.D_l  SaturateOnIntegerOverflow=on  OutDataTypeStr=Inherit: Same as input  ParamDataTypeStr=Inherit: Same as input
  Sim.Nu_r_D_l : Constant  Value=Sim.Nu_r_D_l
  Switch : Switch  Criteria=u2 > Threshold  SaturateOnIntegerOverflow=on
  D_l*Nu_r : Outport
  wires:
  D_l/1 -> Include D_l/1
  Include D_l/1 -> D_l*Nu_r/1
  Switch/1 -> D_l/1
  Nu_r/1 -> Switch/1
  Nu/1 -> Switch/3
  Sim.Nu_r_D_l/1 -> Switch/2

== system sim_4_newnew/Vessel Dynamics1/Vessel LF 6DOF/G ==
  note: G
      | Standard restoring matrix. This effect can
      | be included/excluded from the Parameters file.
      | OS2002
  Eta : Inport
  G : Gain  Gain=Par.Vessel.G  Multiplication=Matrix(K*u)  SaturateOnIntegerOverflow=on  OutDataTypeStr=Inherit: Same as input  ParamDataTypeStr=Inherit: Same as input
  Include G : Gain  Gain=Sim.G  SaturateOnIntegerOverflow=on  OutDataTypeStr=Inherit: Same as input  ParamDataTypeStr=Inherit: Same as input
  G*Eta : Outport
  wires:
  Eta/1 -> G/1
  G/1 -> Include G/1
  Include G/1 -> G*Eta/1

== system sim_4_newnew/Vessel Dynamics1/Vessel LF 6DOF/J(Eta) ==
  note: Theta
  note: v
  note: omega
  note: J(Eta)
      | Standard 6DOF rotation matrix, as defined by Fossen. Using the two
      | rotation matrices Rnb and Tnb from the gnc Simulink toolbox.
      | OS2002
  Eta : Inport
  Nu : Inport  Port=2
  Mux : Mux  Inputs=2
  Product : Product  Inputs=**  Multiplication=Matrix(*)  SaturateOnIntegerOverflow=on  OutDataTypeStr=Inherit: Same as first input
  Product1 : Product  Inputs=**  Multiplication=Matrix(*)  SaturateOnIntegerOverflow=on  OutDataTypeStr=Inherit: Same as first input
  Rnb_gnc : Subsystem
  Selector : Selector  InputPortWidth=6  IndexOptions=Index vector (dialog)  Indices=[4 5 6]  OutputSizes=1
  Selector1 : Selector  InputPortWidth=6  IndexOptions=Index vector (dialog)  Indices=[1 2 3]  OutputSizes=1
  Selector2 : Selector  InputPortWidth=6  IndexOptions=Index vector (dialog)  Indices=[4 5 6]  OutputSizes=1
  Tnb_gnc : Subsystem
  Eta_dot : Outport
  wires:
  Selector/1 -> Tnb_gnc/1(theta), Rnb_gnc/1(theta)
  Eta/1 -> Selector/1
  Rnb_gnc/1(Rzyx) -> Product/1
  Nu/1 -> Selector1/1, Selector2/1
  Selector1/1 -> Product/2
  Selector2/1 -> Product1/2
  Tnb_gnc/1(T) -> Product1/1
  Product/1 -> Mux/1
  Mux/1 -> Eta_dot/1
  Product1/1 -> Mux/2

== system sim_4_newnew/Vessel Dynamics1/Vessel LF 6DOF/Rel velocity ==
  note: REL VELOCITY
      | Calculate relative vessel velociy
      | including current.
      | OS2002
  Nu : Inport
  Current : Inport  Port=2
  Mux : Mux  Inputs=2
  Sum : Sum  Inputs=+-  SaturateOnIntegerOverflow=on
  Zeros : Constant  Value=[0 0 0 0]
  Nu_r : Outport
  wires:
  Current/1 -> Mux/1
  Nu/1 -> Sum/1
  Sum/1 -> Nu_r/1
  Mux/1 -> Sum/2
  Zeros/1 -> Mux/2

== system sim_4_newnew/Vessel Dynamics1/Vessel LF 6DOF/Rotate_yaw_T ==
  note: ROTATE_YAW_T
      | The transposed rotation matrix in yaw, as defined
      | by Fossen. Rotates a velocity or coordinate a positive
      | yaw angle. Corresponds to matlab function  rotate_yaw_T
      | by OS. Uses the gcn Simulink function GNC: "Transposed
      | rotation matrix yaw"
      | OS2002
  Eta : Inport
  nu_2D_NED : Inport  Port=2
  "GNC: \"Transposed rotation matrix yaw\"" : Subsystem
  Mux : Mux  Inputs=2
  Selector : Selector  InputPortWidth=3  IndexOptions=Index vector (dialog)  Indices=[1 2]  OutputSizes=1
  Selector1 : Selector  InputPortWidth=6  IndexOptions=Index vector (dialog)  Indices=6  OutputSizes=1
  psi : Constant  Value=0
  nu_2D_body : Outport
  wires:
  Selector1/1 -> "GNC: \"Transposed rotation matrix yaw\""/1(psi)
  nu_2D_NED/1 -> Mux/1
  psi/1 -> Mux/2
  "GNC: \"Transposed rotation matrix yaw\""/1(R*nu) -> Selector/1
  Selector/1 -> nu_2D_body/1
  Eta/1 -> Selector1/1
  Mux/1 -> "GNC: \"Transposed rotation matrix yaw\""/2(nu)

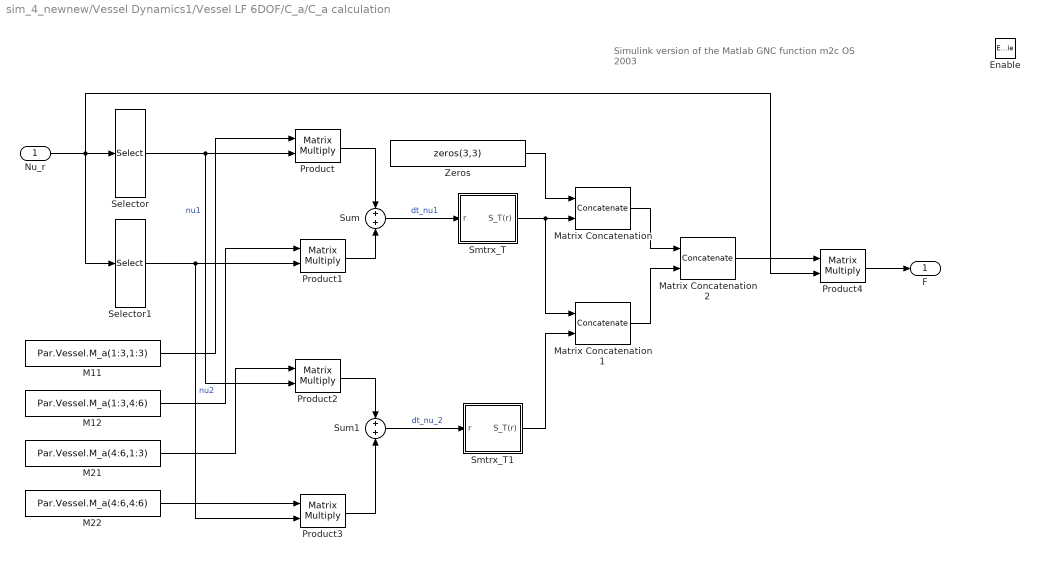
== system sim_4_newnew/Vessel Dynamics1/Vessel LF 6DOF/C_a/C_a calculation ==
  note: Simulink version of the Matlab GNC function m2c
      | OS 2003
  Nu_r : Inport
  Enable : EnablePort
  M11 : Constant  Value=Par.Vessel.M_a(1:3,1:3)
  M12 : Constant  Value=Par.Vessel.M_a(1:3,4:6)
  M21 : Constant  Value=Par.Vessel.M_a(4:6,1:3)
  M22 : Constant  Value=Par.Vessel.M_a(4:6,4:6)
  Matrix Concatenation : Concatenate  Mode=Multidimensional array  ConcatenateDimension=2
  Matrix Concatenation1 : Concatenate  Mode=Multidimensional array  ConcatenateDimension=2
  Matrix Concatenation2 : Concatenate  Mode=Multidimensional array
  Product{,1..4} (5 alike) : Product  Multiplication=Matrix(*)  SaturateOnIntegerOverflow=on  OutDataTypeStr=Inherit: Same as first input
  Selector : Selector  InputPortWidth=6  IndexOptions=Index vector (dialog)  Indices=[1:3]  OutputSizes=1
  Selector1 : Selector  InputPortWidth=6  IndexOptions=Index vector (dialog)  Indices=[4:6]  OutputSizes=1
  Smtrx_T : Subsystem
  Smtrx_T1 : Subsystem
  Sum : Sum  Inputs=+|+  SaturateOnIntegerOverflow=on
  Sum1 : Sum  Inputs=+|+  SaturateOnIntegerOverflow=on
  Zeros : Constant  Value=zeros(3,3)
  F : Outport
  wires:
  Nu_r/1 -> Selector/1, Selector1/1, Product4/2
  Product/1 -> Sum/1
  Product1/1 -> Sum/2
  Product2/1 -> Sum1/1
  Product3/1 -> Sum1/2
  Sum/1 -> Smtrx_T/1(r)  "dt_nu1"
  Sum1/1 -> Smtrx_T1/1(r)  "dt_nu_2"
  Zeros/1 -> Matrix Concatenation/1
  Smtrx_T/1(S_T(r)) -> Matrix Concatenation/2, Matrix Concatenation1/1
  Smtrx_T1/1(S_T(r)) -> Matrix Concatenation1/2
  Matrix Concatenation/1 -> Matrix Concatenation2/1
  Matrix Concatenation1/1 -> Matrix Concatenation2/2
  Product4/1 -> F/1
  Selector/1 -> Product/2, Product2/2  "nu1"
  Selector1/1 -> Product1/2, Product3/2  "nu2"
  M11/1 -> Product/1
  M12/1 -> Product1/1
  M22/1 -> Product3/1
  M21/1 -> Product2/1
  Matrix Concatenation2/1 -> Product4/1

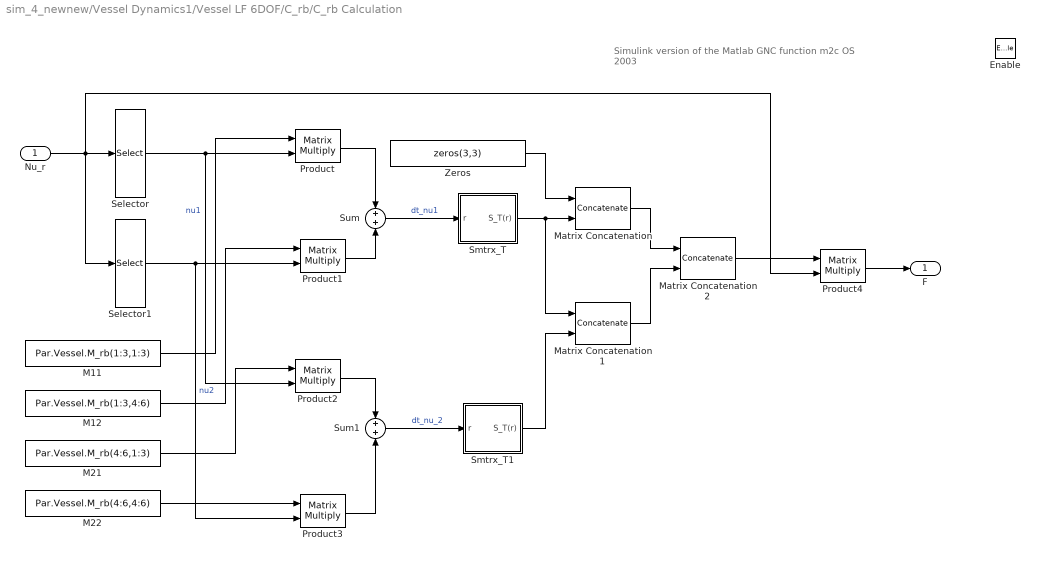
== system sim_4_newnew/Vessel Dynamics1/Vessel LF 6DOF/C_rb/C_rb Calculation ==
  note: Simulink version of the Matlab GNC function m2c
      | OS 2003
  Nu_r : Inport
  Enable : EnablePort
  M11 : Constant  Value=Par.Vessel.M_rb(1:3,1:3)
  M12 : Constant  Value=Par.Vessel.M_rb(1:3,4:6)
  M21 : Constant  Value=Par.Vessel.M_rb(4:6,1:3)
  M22 : Constant  Value=Par.Vessel.M_rb(4:6,4:6)
  Matrix Concatenation : Concatenate  Mode=Multidimensional array  ConcatenateDimension=2
  Matrix Concatenation1 : Concatenate  Mode=Multidimensional array  ConcatenateDimension=2
  Matrix Concatenation2 : Concatenate  Mode=Multidimensional array
  Product{,1..4} (5 alike) : Product  Multiplication=Matrix(*)  SaturateOnIntegerOverflow=on  OutDataTypeStr=Inherit: Same as first input
  Selector : Selector  InputPortWidth=6  IndexOptions=Index vector (dialog)  Indices=[1:3]  OutputSizes=1
  Selector1 : Selector  InputPortWidth=6  IndexOptions=Index vector (dialog)  Indices=[4:6]  OutputSizes=1
  Smtrx_T : Subsystem
  Smtrx_T1 : Subsystem
  Sum : Sum  Inputs=+|+  SaturateOnIntegerOverflow=on
  Sum1 : Sum  Inputs=+|+  SaturateOnIntegerOverflow=on
  Zeros : Constant  Value=zeros(3,3)
  F : Outport
  wires:
  Nu_r/1 -> Selector/1, Selector1/1, Product4/2
  Product/1 -> Sum/1
  Product1/1 -> Sum/2
  Product2/1 -> Sum1/1
  Product3/1 -> Sum1/2
  Sum/1 -> Smtrx_T/1(r)  "dt_nu1"
  Sum1/1 -> Smtrx_T1/1(r)  "dt_nu_2"
  Zeros/1 -> Matrix Concatenation/1
  Smtrx_T/1(S_T(r)) -> Matrix Concatenation/2, Matrix Concatenation1/1
  Smtrx_T1/1(S_T(r)) -> Matrix Concatenation1/2
  Matrix Concatenation/1 -> Matrix Concatenation2/1
  Matrix Concatenation1/1 -> Matrix Concatenation2/2
  Product4/1 -> F/1
  Selector/1 -> Product/2, Product2/2  "nu1"
  Selector1/1 -> Product1/2, Product3/2  "nu2"
  M11/1 -> Product/1
  M12/1 -> Product1/1
  M22/1 -> Product3/1
  M21/1 -> Product2/1
  Matrix Concatenation2/1 -> Product4/1

== system sim_4_newnew/Vessel Dynamics1/Vessel LF 6DOF/J(Eta)/Rnb_gnc ==
  note: gnc Simulink toolbox
  theta : Inport
  Mux2 : Mux  Inputs=2
  Mux3 : Mux  Inputs=9
  R11 : Fcn  Expr=u(6)*u(5)
  R12 : Fcn  Expr=u(6)*u(2)*u(1)-u(3)*u(4)
  R13 : Fcn  Expr=u(4)*u(2)*u(6)+u(3)*u(1)
  "R21 " : Fcn  Expr=u(3)*u(5)
  R22 : Fcn  Expr=u(3)*u(2)*u(1)+u(6)*u(4)
  R23 : Fcn  Expr=u(3)*u(2)*u(4)-u(6)*u(1)
  "R31 " : Fcn  Expr=-u(2)
  R32 : Fcn  Expr=u(5)*u(1)
  R33 : Fcn  Expr=u(5)*u(4)
  Reshape 9x1->3x3 : Reshape  OutputDimensionality=Customize  OutputDimensions=[3,3]
  cos(theta) : Trigonometry  Operator=cos
  sin(theta) : Trigonometry
  Rzyx : Outport  InitialOutput=0
  wires:
  R11/1 -> Mux3/1
  Mux3/1 -> Reshape 9x1->3x3/1
  Reshape 9x1->3x3/1 -> Rzyx/1
  sin(theta)/1 -> Mux2/1
  cos(theta)/1 -> Mux2/2
  theta/1 -> cos(theta)/1, sin(theta)/1
  Mux2/1 -> R32/1, R13/1, R33/1, R23/1, R22/1, "R31 "/1, R11/1, "R21 "/1, R12/1
  R23/1 -> Mux3/8
  R13/1 -> Mux3/7
  R22/1 -> Mux3/5
  R12/1 -> Mux3/4
  "R31 "/1 -> Mux3/3
  "R21 "/1 -> Mux3/2
  R32/1 -> Mux3/6
  R33/1 -> Mux3/9
